simulink model "PID_GuidageLateral_2015"  (R2015b)
settings: Solver=ode45  SolverMode=SingleTasking  StartTime=0.0  StopTime=240  RelTol=1e-3
values from neighbouring files (symbols this model uses):
  DEG2RAD = pi/180.    (= 0.0174532925199)    [main.m]
  g = 9.80665    [main.m]
  gammae = 0*DEG2RAD    (= 0)    [main.m]
  k1 = Vp/(g*nze*tauCap)    [main.m]
  k2 = Vp/(g*nze*tauCap*tauEy)    [main.m]
  KTS2MS = 1852. / 3600.    (= 0.514444444444)    [main.m]
  NM2M = 1852.    (= 1852)    [main.m]
  phiMax = 30*DEG2RAD    (= 0.523598775598)    [main.m]
  psiW = 90*DEG2RAD    (= 1.57079632679)    [main.m]
  tauEy = 4*tauCap    (= 60)    [main.m]
  Ve = 180*KTS2MS    (= 92.6)    [main.m]
  Vp = Ve*cos(gammae)    [main.m]
  W = 1*50*KTS2MS    (= 25.7222222222)    [main.m]
undefined symbols (not defined in the file or in its folder): chi_c, chi_e, dirAxe, xAxe, yAxe
settings Model: Creator=miquelth  LastModifiedBy=miquelth
settings DataIOCC: LimitDataPoints=off  ReturnWorkspaceOutputs=on
settings DebuggingCC: SFUnexpectedBacktrackingDiag=error  SFNoUnconditionalDefaultTransitionDiag=error
settings HardwareCC: ProdWordSize=32  ProdHWDeviceType=Specified
settings ModelReferenceCC: PropagateSignalLabelsOutOfModel=on
settings SFSimCC: SimUseLocalCustomCode=on
settings RTWCC: RTWUseLocalCustomCode=on
settings GRTTargetCC: TargetLangStandard=C99 (ISO)
settings ConfigComp: CovMetricSettings=dwe  CovHtmlReporting=off  CovSaveCumulativeToWorkspaceVar=off  CovSaveSingleToWorkspaceVar=off  CovModelRefEnable=Off  CovExternalEMLEnable=on

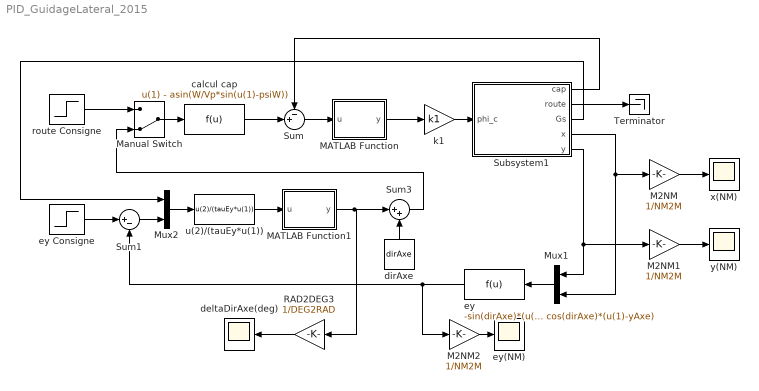
== system PID_GuidageLateral_2015 ==
  M2NM : Gain  Gain=1/NM2M
  M2NM1 : Gain  Gain=1/NM2M
  M2NM2 : Gain  Gain=1/NM2M
  MATLAB Function : MATLAB Function  TreatAsAtomicUnit=on
  MATLAB Function1 : MATLAB Function  TreatAsAtomicUnit=on
  Manual Switch : ManualSwitch  CurrentSetting=0
  Mux1 : Mux  Inputs=2
  Mux2 : Mux  Inputs=2
  RAD2DEG3 : Gain  Gain=1/DEG2RAD
  Subsystem1 : Subsystem
  Sum : Sum  Inputs=-+|
  Sum1 : Sum  Inputs=|+-
  Sum3 : Sum  Inputs=|++
  Terminator : Terminator
  calcul cap : Fcn  Expr=u(1) - asin(W/Vp*sin(u(1)-psiW))
  deltaDirAxe(deg) : Scope
  dirAxe : Constant  Value=dirAxe
  ey : Fcn  Expr=-sin(dirAxe)*(u(2)-xAxe) + cos(dirAxe)*(u(1)-yAxe)
  ey Consigne : Step  Time=0  After=0  SampleTime=0
  ey(NM) : Scope
  k1 : Gain  Gain=k1
  route Consigne : Step  Time=0  Before=chi_e  After=chi_c  SampleTime=0
  u(2)/(tauEy*u(1)) : Fcn  Expr=u(2)/(tauEy*u(1))
  x(NM) : Scope
  y(NM) : Scope
  wires:
  Sum/1 -> MATLAB Function/1(u)
  MATLAB Function/1(y) -> k1/1
  calcul cap/1 -> Sum/2
  Subsystem1/1(cap) -> Sum/1
  k1/1 -> Subsystem1/1(phi_c)
  ey Consigne/1 -> Sum1/1
  Mux1/1 -> ey/1
  Subsystem1/4(x) -> M2NM/1, Mux1/2
  Sum1/1 -> Mux2/2
  Subsystem1/3(Gs) -> Mux2/1
  Mux2/1 -> u(2)/(tauEy*u(1))/1
  M2NM/1 -> x(NM)/1
  Subsystem1/5(y) -> M2NM1/1, Mux1/1
  M2NM1/1 -> y(NM)/1
  ey/1 -> M2NM2/1, Sum1/2
  M2NM2/1 -> ey(NM)/1
  RAD2DEG3/1 -> deltaDirAxe(deg)/1
  Manual Switch/1 -> calcul cap/1
  route Consigne/1 -> Manual Switch/1
  u(2)/(tauEy*u(1))/1 -> MATLAB Function1/1(u)
  MATLAB Function1/1(y) -> RAD2DEG3/1, Sum3/1
  dirAxe/1 -> Sum3/2
  Sum3/1 -> Manual Switch/2
  Subsystem1/2(route) -> Terminator/1

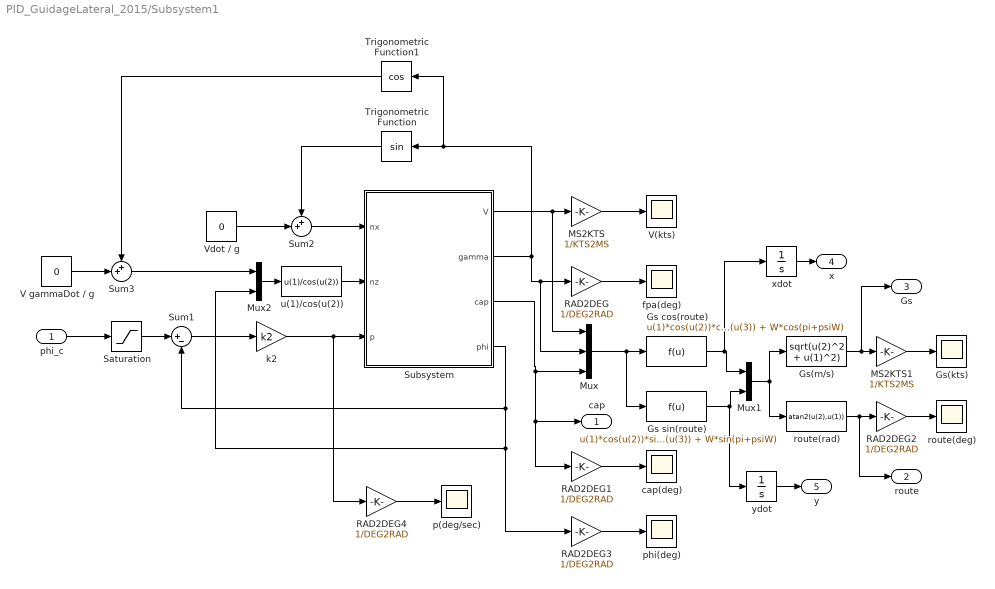
== system PID_GuidageLateral_2015/Subsystem1 ==
  phi_c : Inport
  Gs cos(route) : Fcn  Expr=u(1)*cos(u(2))*cos(u(3)) + W*cos(pi+psiW)
  Gs sin(route) : Fcn  Expr=u(1)*cos(u(2))*sin(u(3)) + W*sin(pi+psiW)
  Gs(kts) : Scope
  Gs(m/s) : Fcn  Expr=sqrt(u(2)^2 + u(1)^2)
  MS2KTS : Gain  Gain=1/KTS2MS
  MS2KTS1 : Gain  Gain=1/KTS2MS
  Mux : Mux  Inputs=3
  Mux1 : Mux  Inputs=2
  Mux2 : Mux  Inputs=2
  RAD2DEG{,1..4} (5 alike) : Gain  Gain=1/DEG2RAD
  Saturation : Saturate  UpperLimit=phiMax  LowerLimit=-phiMax
  Subsystem : Subsystem
  Sum1 : Sum  Inputs=|+-
  Sum2 : Sum  Inputs=++|
  Sum3 : Sum  Inputs=++|
  Trigonometric Function : Trigonometry
  Trigonometric Function1 : Trigonometry  Operator=cos
  V gammaDot / g : Constant  Value=0
  V(kts) : Scope
  Vdot / g : Constant  Value=0
  cap(deg) : Scope
  fpa(deg) : Scope
  k2 : Gain  Gain=k2
  p(deg/sec) : Scope
  phi(deg) : Scope
  route(deg) : Scope
  route(rad) : Fcn  Expr=atan2(u(2),u(1))
  u(1)/cos(u(2)) : Fcn  Expr=u(1)/cos(u(2))
  xdot : Integrator
  ydot : Integrator
  cap : Outport
  route : Outport  Port=2
  Gs : Outport  Port=3
  x : Outport  Port=4
  y : Outport  Port=5
  wires:
  Saturation/1 -> Sum1/1
  Sum1/1 -> k2/1
  k2/1 -> RAD2DEG4/1, Subsystem/3(p)
  phi_c/1 -> Saturation/1
  Subsystem/3(cap) -> cap/1, RAD2DEG1/1, Mux/3
  Subsystem/1(V) -> Mux/1, MS2KTS/1
  Subsystem/2(gamma) -> Mux/2, RAD2DEG/1, Trigonometric Function1/1, Trigonometric Function/1
  MS2KTS/1 -> V(kts)/1
  RAD2DEG/1 -> fpa(deg)/1
  Mux/1 -> Gs sin(route)/1, Gs cos(route)/1
  RAD2DEG1/1 -> cap(deg)/1
  Gs cos(route)/1 -> xdot/1, Mux1/1
  Gs sin(route)/1 -> ydot/1, Mux1/2
  Mux1/1 -> route(rad)/1, Gs(m/s)/1
  Gs(m/s)/1 -> Gs/1, MS2KTS1/1
  MS2KTS1/1 -> Gs(kts)/1
  route(rad)/1 -> route/1, RAD2DEG2/1
  RAD2DEG2/1 -> route(deg)/1
  Subsystem/4(phi) -> Sum1/2, Mux2/2, RAD2DEG3/1
  RAD2DEG3/1 -> phi(deg)/1
  Vdot / g/1 -> Sum2/2
  Trigonometric Function/1 -> Sum2/1
  Sum2/1 -> Subsystem/1(nx)
  V gammaDot / g/1 -> Sum3/2
  Trigonometric Function1/1 -> Sum3/1
  Mux2/1 -> u(1)/cos(u(2))/1
  u(1)/cos(u(2))/1 -> Subsystem/2(nz)
  Sum3/1 -> Mux2/1
  RAD2DEG4/1 -> p(deg/sec)/1
  xdot/1 -> x/1
  ydot/1 -> y/1

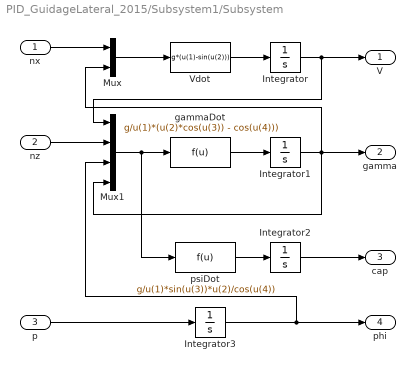
== system PID_GuidageLateral_2015/Subsystem1/Subsystem ==
  nx : Inport
  nz : Inport  Port=2
  p : Inport  Port=3
  Integrator : Integrator  InitialCondition=Ve
  Integrator1 : Integrator  InitialCondition=gammae
  Integrator2 : Integrator
  Integrator3 : Integrator
  Mux : Mux  Inputs=2
  Mux1 : Mux
  Vdot : Fcn  Expr=g*(u(1)-sin(u(2)))
  gammaDot : Fcn  Expr=g/u(1)*(u(2)*cos(u(3)) - cos(u(4)))
  psiDot : Fcn  Expr=g/u(1)*sin(u(3))*u(2)/cos(u(4))
  V : Outport
  gamma : Outport  Port=2
  cap : Outport  Port=3
  phi : Outport  Port=4
  wires:
  Mux/1 -> Vdot/1
  nz/1 -> Mux1/2
  Vdot/1 -> Integrator/1
  Integrator/1 -> V/1, Mux1/1
  Mux1/1 -> psiDot/1, gammaDot/1
  gammaDot/1 -> Integrator1/1
  Integrator1/1 -> gamma/1, Mux1/4, Mux/2
  psiDot/1 -> Integrator2/1
  Integrator2/1 -> cap/1
  nx/1 -> Mux/1
  p/1 -> Integrator3/1
  Integrator3/1 -> phi/1, Mux1/3

== matlab function PID_GuidageLateral_2015/MATLAB Function1 ==
  data: u input; y output
function y = fcn(u)
    y = u;
    while y > pi
        y = y-2*pi
    end
    while y < -pi
        y = y+2*pi
    end
    %limitation de l'angle de convergence
    DEG2RAD = pi/180;
    deltaDirMax = 45*DEG2RAD; 
    if y > deltaDirMax
        y = deltaDirMax;
    elseif y < -deltaDirMax
        y = -deltaDirMax;
    end
end

== matlab function PID_GuidageLateral_2015/MATLAB Function ==
  data: u input; y output
function y = fcn(u)
    y = u;
    while y > pi
        y = y-2*pi
    end
    while y < -pi
        y = y+2*pi
    end
end
